simulink model "Dynamics_SIM"  (R2025b)
settings: Solver=FixedStepAuto  StartTime=0.0  StopTime=tspan  FixedStep=dt_sim  RelTol=rel_tol  AbsTol=abs_tol
undefined symbols (not defined in the file): test_ft_list, test_pwm_list
settings Model: SimulationMode=accelerator  Creator=koryh  LastModifiedBy=matthewlin

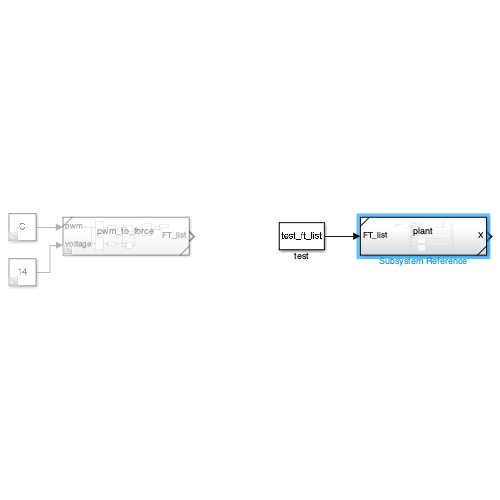
[thumbnail: Simulink's stored preview of the top-level diagram]
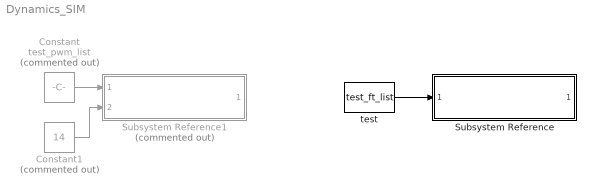
== system Dynamics_SIM ==
  Constant : Constant  Commented=on  Value=test_pwm_list
  Constant1 : Constant  Commented=on  Value=14
  Subsystem Reference : Subsystem  ReferencedSubsystem=plant
  Subsystem Reference1 : Subsystem  Commented=on  ReferencedSubsystem=pwm_to_force
  test : Constant  Value=test_ft_list
  wires:
  Constant/1 -> Subsystem Reference1/1
  Constant1/1 -> Subsystem Reference1/2
  test/1 -> Subsystem Reference/1
